simulink model "simQuadrotor"  (R2014b)
settings: Solver=ode45  StartTime=0.0  StopTime=tof  FixedStep=dt  MaxStep=dtmax  RelTol=1e-3
values from neighbouring files (symbols this model uses):
  a = (IzzT - IxxT)./ IxxT    [quadrotor.m]
  alpha = 1    [quadrotor.m]
  Aq = -20    [quadrotor.m]
  Ar = -10*eye(2)    [quadrotor.m]
  Arm = [-20 0 ; 0 -5]    [quadrotor.m]
  As = -50*eye(3)    [quadrotor.m]
  attitudeControlFlag = 4    [quadrotor.m]
  Bq = 1    [quadrotor.m]
  Br = [1 0]    [quadrotor.m]
  Dhat0 = zeros(3,1)    [quadrotor.m]
  Dlimit = 2.5    [quadrotor.m]
  DSecondLimit = 2    [quadrotor.m]
  dtFc = 10e-3    (= 0.01)    [quadrotor.m]
  epsilon = 0.1    [quadrotor.m]
  epsilontheta = 0.1    [quadrotor.m]
  euler0 = [0 0 0]'*pi/180    [quadrotor.m]
  Eulerc_ftc = [0 0 0]'    [quadrotor.m]
  faultyPropellerVec = double(not(faultyPropellerVec))    [quadrotor.m]
  FDstart = 3    [quadrotor.m]
  flims = [0.2*0 3.8*2.5]    [quadrotor.m]
  ftc_f2 = 0.1*2    (= 0.2)    [quadrotor.m]
  g = 9.81    [quadrotor.m]
  GammaW = 10000    [quadrotor.m]
  IxxB = IxxT - 4*IxxP    (= 0.0027)    [quadrotor.m]
  IxxT = 2.7e-3    (= 0.0027)    [quadrotor.m]
  IyyB = IyyT - 4*IyyP    (= 0.0027)    [quadrotor.m]
  IyyT = IxxT    (= 0.0027)    [quadrotor.m]
  IzzB = IzzT - 4*IzzP    (= 0.00514)    [quadrotor.m]
  IzzP = 1.5e-5    (= 1.5e-05)    [quadrotor.m]
  IzzT = 5.2e-3    (= 0.0052)    [quadrotor.m]
  Kdxx = 0.7e-4/10    (= 7e-06)    [quadrotor.m]
  Kdzz = 1.4e-4    (= 0.00014)    [quadrotor.m]
  Kf = 6.41e-6    (= 6.41e-06)    [quadrotor.m]
  Kp = 2*0.75*diag([1 1 1])    [quadrotor.m]
  Kp4 = 0.05    [quadrotor.m]
  Ktau = 1.72e-2    (= 0.0172)    [quadrotor.m]
  Kv = 0*0.005*diag([1 1 1])    [quadrotor.m]
  Kv4 = 0.02    [quadrotor.m]
  l = 0.17    [quadrotor.m]
  m = 0.5    [quadrotor.m]
  nc_ftc = 1    [quadrotor.m]
  nCheby = 3    [quadrotor.m]
  pqr0 = [0 0 0]'*pi/180    [quadrotor.m]
  Ps = lyap(As',Q)    [quadrotor.m]
  q0 = [euler0 ; pqr0]    [quadrotor.m]
  qp0 = 0    [quadrotor.m]
  sigmaMot = 0.015    [quadrotor.m]
  tfault = 5    [quadrotor.m]
  Vb0 = [0 0 0]'    [quadrotor.m]
  W0 = 0    [quadrotor.m]
  Wbnd = 10    [quadrotor.m]
  Xe0 = [0 0 0]'    [quadrotor.m]
  xhat0 = [pqr0]    [quadrotor.m]
undefined symbols (not defined in the file or in its folder): Intmax, Intmin, magnitude, rmax, rmin
libraries: aerolibutil x38, simulink x11, vrlib x3, dspbuff3 x1
(part 3 of 3)

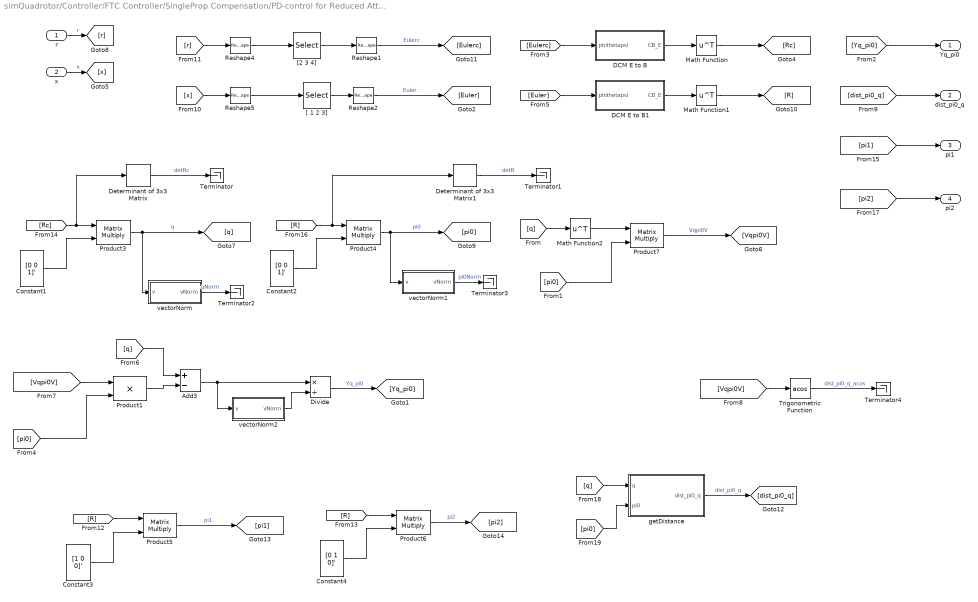
== system simQuadrotor/Controller/FTC Controller/SingleProp Compensation/PD-control for Reduced Attitude-Bullo/getRedAttRelatedPars ==
  r : Inport
  x : Inport  Port=2
  Add3 : Sum  Inputs=+-
  Constant1 : Constant  Value=[0 0 1]'  VectorParams1D=off
  Constant2 : Constant  Value=[0 0 1]'  VectorParams1D=off
  Constant3 : Constant  Value=[1 0 0]'  VectorParams1D=off
  Constant4 : Constant  Value=[0 1 0]'  VectorParams1D=off
  DCM E to B : Subsystem
  DCM E to B1 : Subsystem
  Determinant of 3x3 Matrix : aerolibutil/Determinant of 3x3 Matrix
  Determinant of 3x3 Matrix1 : aerolibutil/Determinant of 3x3 Matrix
  Divide : Product  Inputs=*/
  Math Function : Math  Operator=transpose  SaturateOnIntegerOverflow=on
  Math Function1 : Math  Operator=transpose  SaturateOnIntegerOverflow=on
  Math Function2 : Math  Operator=transpose  SaturateOnIntegerOverflow=on
  Product1 : Product  RndMeth=Zero
  Product{3..7} (5 alike) : Product  Multiplication=Matrix(*)  RndMeth=Zero
  Reshape{1..2,4..5} (4 alike) : Reshape  OutputDimensionality=Column vector (2-D)
  Terminator{,1..4} (5 alike) : Terminator
  Trigonometric Function : Trigonometry  Operator=acos
  "[ 1 2 3]" : Selector  NumberOfDimensions=2  InputPortWidth=3  IndexOptions=Index vector (dialog),Index vector (dialog)  Indices=[1 2 3],1  OutputSizes=1,1
  "[2 3 4]" : Selector  NumberOfDimensions=2  InputPortWidth=3  IndexOptions=Index vector (dialog),Index vector (dialog)  Indices=[2 3 4],1  OutputSizes=1,1
  getDistance : Subsystem
  vectorNorm : Subsystem
  vectorNorm1 : Subsystem
  vectorNorm2 : Subsystem
  Yq_pi0 : Outport
  dist_pi0_q : Outport  Port=2
  pi1 : Outport  Port=3
  pi2 : Outport  Port=4
  wires:
  [pi0] -> getDistance/2(pi0)
  [q] -> getDistance/1(q)
  getDistance/1(dist_pi0_q) -> [dist_pi0_q]  "dist_pi0_q"
  vectorNorm1/1(vNorm) -> Terminator3/1  "pi0Norm"
  vectorNorm/1(vNorm) -> Terminator2/1  "qNorm"
  Determinant of 3x3 Matrix1/1 -> Terminator1/1  "detR"
  Determinant of 3x3 Matrix/1 -> Terminator/1  "detRc"
  [pi2] -> pi2/1
  [pi1] -> pi1/1
  [R] -> Product6/1
  Constant4/1 -> Product6/2
  Product6/1 -> [pi2]  "pi2"
  [R] -> Product5/1
  Constant3/1 -> Product5/2
  Product5/1 -> [pi1]  "pi1"
  [Yq_pi0] -> Yq_pi0/1
  Trigonometric Function/1 -> Terminator4/1  "dist_pi0_q_acos"
  [Vqpi0V] -> Trigonometric Function/1
  [Vqpi0V] -> Product1/1
  Product7/1 -> [Vqpi0V]  "Vqpi0V"
  Divide/1 -> [Yq_pi0]  "Yq_pi0"
  vectorNorm2/1(vNorm) -> Divide/2
  Add3/1 -> Divide/1, vectorNorm2/1(v)
  Product1/1 -> Add3/2
  [q] -> Add3/1
  [pi0] -> Product1/2
  [pi0] -> Product7/2
  Math Function2/1 -> Product7/1
  [q] -> Math Function2/1
  [dist_pi0_q] -> dist_pi0_q/1
  [Rc] -> Product3/1, Determinant of 3x3 Matrix/1
  Constant1/1 -> Product3/2
  Product3/1 -> [q], vectorNorm/1(v)  "q"
  [R] -> Product4/1, Determinant of 3x3 Matrix1/1
  Constant2/1 -> Product4/2
  Product4/1 -> [pi0], vectorNorm1/1(v)  "pi0"
  r/1 -> [r]  "r"
  x/1 -> [x]  "x"
  Math Function1/1 -> [R]
  [x] -> Reshape5/1
  Math Function/1 -> [Rc]
  "[ 1 2 3]"/1 -> Reshape2/1
  Reshape5/1 -> "[ 1 2 3]"/1
  Reshape2/1 -> [Euler]  "Euler"
  Reshape1/1 -> [Eulerc]  "Eulerc"
  "[2 3 4]"/1 -> Reshape1/1
  [r] -> Reshape4/1
  [Eulerc] -> DCM E to B/1(phithetapsi)
  DCM E to B/1(CB_E) -> Math Function/1
  Reshape4/1 -> "[2 3 4]"/1
  [Euler] -> DCM E to B1/1(phithetapsi)
  DCM E to B1/1(CB_E) -> Math Function1/1

== system simQuadrotor/Controller/FTC Controller/SingleProp Compensation/Perturbation Calculation/Reference model ==
  x1 : Inport
  Gain : Gain  Gain=Arm  Multiplication=Matrix(K*u)
  f1r : Outport
  wires:
  Gain/1 -> [f1r]
  x1/1 -> [x1]
  [x1] -> Gain/1
  [f1r] -> f1r/1

== system simQuadrotor/Controller/FTC Controller/SingleProp Compensation/Perturbation Calculation/System model ==
  x1 : Inport
  w3 : Inport  Port=2
  r : Inport  Port=3
  p1p : Inport  Port=4
  p2p : Inport  Port=5
  Add2 : Sum  Inputs=+++
  Constant : Constant  Value=a  VectorParams1D=off
  Constant1 : Constant  Value=Br  VectorParams1D=off
  Constant2 : Constant  Value=ftc_f2  VectorParams1D=off
  Constant3 : Constant  Value=[0 0]'  VectorParams1D=off
  Constant5 : Constant  Value=0  VectorParams1D=off
  Gain : Gain  Gain=-1
  Gain1 : Gain
  Gain2 : Gain  Gain=l/IxxT
  Gain3 : Gain  Gain=[0 ; 1]  Multiplication=Matrix(K*u)
  Gain4 : Gain  Gain=-1
  Mux : Mux  Inputs=2
  Product1 : Product  Multiplication=Matrix(*)
  Product2 : Product
  Product3 : Product  Multiplication=Matrix(*)
  Product4 : Product  Multiplication=Matrix(*)
  Reshape : Reshape  OutputDimensionality=Customize  OutputDimensions=[2,2]
  Reshape3 : Reshape  OutputDimensionality=Column vector (2-D)
  Vector Concatenate : Concatenate  NumInputs=3
  f1 : Outport
  wires:
  Constant5/1 -> Vector Concatenate/3
  Gain1/1 -> Vector Concatenate/2
  Vector Concatenate/1 -> Reshape/1
  [p2p] -> Gain1/1
  Constant3/1 -> Vector Concatenate/1
  p2p/1 -> [p2p]
  p1p/1 -> [p1p]
  Product4/1 -> Add2/2
  Product3/1 -> Add2/1
  [r] -> Product4/2
  Product1/1 -> Product4/1
  [Br] -> Product1/2
  Reshape3/1 -> Product1/1
  [x1] -> Product3/2
  Reshape/1 -> Product3/1
  [p1p] -> Gain4/1
  Mux/1 -> Reshape3/1
  Constant1/1 -> [Br]
  w3/1 -> [w3]
  r/1 -> [r]
  [a] -> Product2/1  "a"
  [w3] -> Product2/2
  Add2/1 -> [f1]
  Product2/1 -> Gain/1  "aw3"
  Constant/1 -> [a]
  x1/1 -> [x1]
  [f1] -> f1/1
  Gain/1 -> Mux/2
  Constant2/1 -> Gain2/1
  Gain2/1 -> Gain3/1
  Gain3/1 -> Add2/3  "d"
  Gain4/1 -> Mux/1

== system simQuadrotor/Controller/FTC Controller/SingleProp Compensation/Perturbation Calculation/getStates ==
  x : Inport
  Constant : Constant  Value=[0 0 1]'  VectorParams1D=off
  Mux : Mux  Inputs=2
  Reshape{1,3..4,6..7} (5 alike) : Reshape  OutputDimensionality=Column vector (2-D)
  "[2 3 4]1" : Selector  InputPortWidth=3
  "[2 3 4]2" : Selector  InputPortWidth=3  Indices=2
  "[2 3 4]3" : Selector  InputPortWidth=3  Indices=3
  "[4 5 6]" : Selector  NumberOfDimensions=2  InputPortWidth=3  IndexOptions=Index vector (dialog),Index vector (dialog)  Indices=[4 5 6],1  OutputSizes=1,1
  calcParameters : Subsystem  TreatAsAtomicUnit=on
  getDistance : Subsystem
  x1 : Outport
  x2 : Outport  Port=2
  w3 : Outport  Port=3
  p1p : Outport  Port=4
  p2p : Outport  Port=5
  wires:
  [p2p] -> p2p/1
  [p1p] -> p1p/1
  "[2 3 4]1"/1 -> Mux/2
  calcParameters/3(p) -> [p]  "p"
  [p] -> getDistance/2(p)
  Constant/1 -> getDistance/1(q)
  getDistance/1(dist) -> [dist]  "dist"
  calcParameters/2(p2p) -> [p2p]  "p2p"
  calcParameters/1(p1p) -> [p1p]  "p1p"
  [x] -> calcParameters/1(x)
  Reshape7/1 -> [w3]
  Reshape6/1 -> [x2]
  Reshape3/1 -> [x1]
  "[2 3 4]3"/1 -> Reshape7/1
  [w] -> "[2 3 4]3"/1
  "[2 3 4]2"/1 -> Reshape6/1
  [w3] -> w3/1
  [w] -> "[2 3 4]2"/1
  Mux/1 -> Reshape3/1
  [dist] -> Mux/1
  [w] -> "[2 3 4]1"/1
  [x2] -> x2/1  "x2"
  [x1] -> x1/1  "x1"
  x/1 -> [x]  "x"
  Reshape1/1 -> [w]  "w"
  "[4 5 6]"/1 -> Reshape1/1
  [x] -> Reshape4/1
  Reshape4/1 -> "[4 5 6]"/1

== system simQuadrotor/Controller/Nominal Controller/PD-Attitude Control with wB_IB/get eR/DCM E to B ==
  phithetapsi : Inport
  Create 3x3 Matrix : aerolibutil/Create 3x3 Matrix
  Fcn11 : Fcn  Expr=u(5)*u(6)
  Fcn12 : Fcn  Expr=u(3)*u(5)
  Fcn13 : Fcn  Expr=-u(2)
  Fcn21 : Fcn  Expr=u(1)*u(2)*u(6)-u(4)*u(3)
  Fcn22 : Fcn  Expr=u(1)*u(2)*u(3)+u(4)*u(6)
  Fcn23 : Fcn  Expr=u(1)*u(5)
  Fcn31 : Fcn  Expr=u(4)*u(2)*u(6)+u(1)*u(3)
  Fcn32 : Fcn  Expr=u(4)*u(2)*u(3)-u(1)*u(6)
  Fcn33 : Fcn  Expr=u(4)*u(5)
  Mux : Mux  Inputs=2
  sincos : Trigonometry  Operator=sincos
  CB_E : Outport
  wires:
  Create 3x3 Matrix/1 -> CB_E/1  "CB_E"
  phithetapsi/1 -> sincos/1  "phithetapsi"
  Fcn33/1 -> Create 3x3 Matrix/9
  Fcn32/1 -> Create 3x3 Matrix/8
  Fcn23/1 -> Create 3x3 Matrix/6
  Fcn22/1 -> Create 3x3 Matrix/5
  Fcn31/1 -> Create 3x3 Matrix/7
  Fcn21/1 -> Create 3x3 Matrix/4
  Fcn13/1 -> Create 3x3 Matrix/3
  Fcn12/1 -> Create 3x3 Matrix/2
  Fcn11/1 -> Create 3x3 Matrix/1
  Mux/1 -> Fcn21/1, Fcn13/1, Fcn12/1, Fcn11/1, Fcn22/1, Fcn23/1, Fcn31/1, Fcn33/1, Fcn32/1
  sincos/2 -> Mux/2
  sincos/1 -> Mux/1

== system simQuadrotor/Controller/Nominal Controller/PD-Attitude Control with wB_IB/get eR/DCM E to B1 ==
  phithetapsi : Inport
  Create 3x3 Matrix : aerolibutil/Create 3x3 Matrix
  Fcn11 : Fcn  Expr=u(5)*u(6)
  Fcn12 : Fcn  Expr=u(3)*u(5)
  Fcn13 : Fcn  Expr=-u(2)
  Fcn21 : Fcn  Expr=u(1)*u(2)*u(6)-u(4)*u(3)
  Fcn22 : Fcn  Expr=u(1)*u(2)*u(3)+u(4)*u(6)
  Fcn23 : Fcn  Expr=u(1)*u(5)
  Fcn31 : Fcn  Expr=u(4)*u(2)*u(6)+u(1)*u(3)
  Fcn32 : Fcn  Expr=u(4)*u(2)*u(3)-u(1)*u(6)
  Fcn33 : Fcn  Expr=u(4)*u(5)
  Mux : Mux  Inputs=2
  sincos : Trigonometry  Operator=sincos
  CB_E : Outport
  wires:
  Create 3x3 Matrix/1 -> CB_E/1  "CB_E"
  phithetapsi/1 -> sincos/1  "phithetapsi"
  Fcn33/1 -> Create 3x3 Matrix/9
  Fcn32/1 -> Create 3x3 Matrix/8
  Fcn23/1 -> Create 3x3 Matrix/6
  Fcn22/1 -> Create 3x3 Matrix/5
  Fcn31/1 -> Create 3x3 Matrix/7
  Fcn21/1 -> Create 3x3 Matrix/4
  Fcn13/1 -> Create 3x3 Matrix/3
  Fcn12/1 -> Create 3x3 Matrix/2
  Fcn11/1 -> Create 3x3 Matrix/1
  Mux/1 -> Fcn21/1, Fcn13/1, Fcn12/1, Fcn11/1, Fcn22/1, Fcn23/1, Fcn31/1, Fcn33/1, Fcn32/1
  sincos/2 -> Mux/2
  sincos/1 -> Mux/1

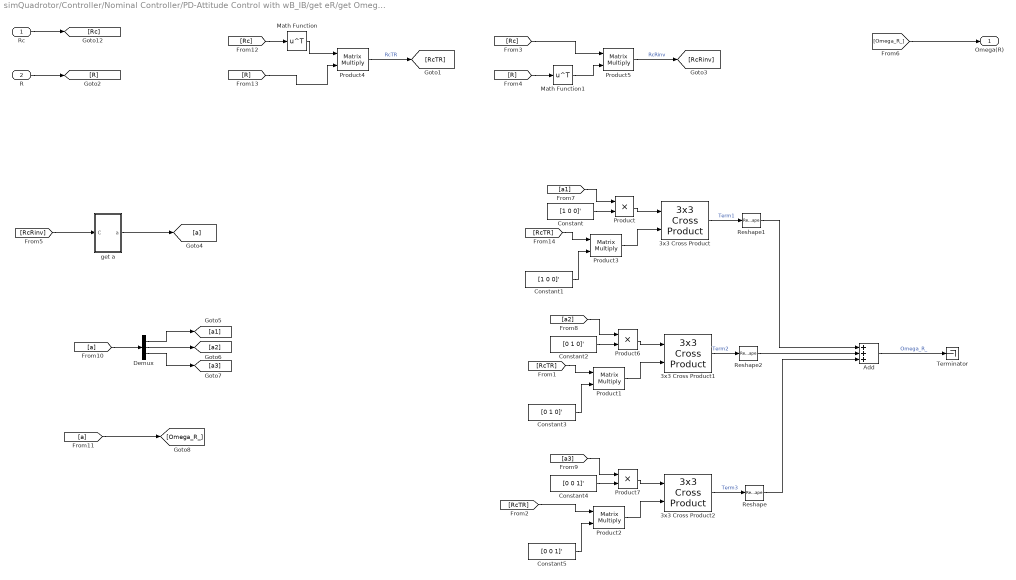
== system simQuadrotor/Controller/Nominal Controller/PD-Attitude Control with wB_IB/get eR/get Omega(R) RBAC ==
  Rc : Inport
  R : Inport  Port=2
  3x3 Cross Product : aerolibutil/3x3 Cross Product
  3x3 Cross Product1 : aerolibutil/3x3 Cross Product
  3x3 Cross Product2 : aerolibutil/3x3 Cross Product
  Add : Sum  Inputs=+++
  Constant : Constant  Value=[1 0 0]'  VectorParams1D=off
  Constant1 : Constant  Value=[1 0 0]'  VectorParams1D=off
  Constant2 : Constant  Value=[0 1 0]'  VectorParams1D=off
  Constant3 : Constant  Value=[0 1 0]'  VectorParams1D=off
  Constant4 : Constant  Value=[0 0 1]'  VectorParams1D=off
  Constant5 : Constant  Value=[0 0 1]'  VectorParams1D=off
  Demux : Demux  Outputs=3
  Math Function : Math  Operator=transpose  SaturateOnIntegerOverflow=on
  Math Function1 : Math  Operator=transpose  SaturateOnIntegerOverflow=on
  Product : Product  RndMeth=Zero
  Product{1..5} (5 alike) : Product  Multiplication=Matrix(*)  RndMeth=Zero
  Product6 : Product  RndMeth=Zero
  Product7 : Product  RndMeth=Zero
  Reshape : Reshape  OutputDimensionality=Column vector (2-D)
  Reshape1 : Reshape  OutputDimensionality=Column vector (2-D)
  Reshape2 : Reshape  OutputDimensionality=Column vector (2-D)
  Terminator : Terminator
  get a : Subsystem
  Omega(R) : Outport
  wires:
  [a] -> [Omega_R_]
  Reshape/1 -> Add/3
  Reshape2/1 -> Add/2
  Reshape1/1 -> Add/1
  Demux/3 -> [a3]
  Demux/2 -> [a2]
  Demux/1 -> [a1]
  [a] -> Demux/1
  [a3] -> Product7/1
  [a2] -> Product6/1
  [a1] -> Product/1
  get a/1(a) -> [a]
  [RcRinv] -> get a/1(C)
  Math Function1/1 -> Product5/2
  Product5/1 -> [RcRinv]  "RcRinv"
  [R] -> Math Function1/1
  [Rc] -> Product5/1
  R/1 -> [R]
  Rc/1 -> [Rc]
  Math Function/1 -> Product4/1
  Product4/1 -> [RcTR]  "RcTR"
  [R] -> Product4/2
  [Rc] -> Math Function/1
  [Omega_R_] -> Omega(R)/1
  Add/1 -> Terminator/1  "Omega_R_"
  3x3 Cross Product2/1 -> Reshape/1  "Term3"
  3x3 Cross Product1/1 -> Reshape2/1  "Term2"
  3x3 Cross Product/1 -> Reshape1/1  "Term1"
  Product7/1 -> 3x3 Cross Product2/1
  Product2/1 -> 3x3 Cross Product2/2
  Constant5/1 -> Product2/2
  [RcTR] -> Product2/1
  Constant4/1 -> Product7/2
  Product6/1 -> 3x3 Cross Product1/1
  Product/1 -> 3x3 Cross Product/1
  Product1/1 -> 3x3 Cross Product1/2
  Constant3/1 -> Product1/2
  [RcTR] -> Product1/1
  Constant2/1 -> Product6/2
  Product3/1 -> 3x3 Cross Product/2
  Constant1/1 -> Product3/2
  [RcTR] -> Product3/1
  Constant/1 -> Product/2

== system simQuadrotor/Controller/Nominal Controller/PD-Attitude Control with wB_IB/get eR/get eR ==
  note: Vee map
  Rc : Inport
  R : Inport  Port=2
  13 : Selector  NumberOfDimensions=2  InputPortWidth=3  IndexOptions=Index vector (dialog),Index vector (dialog)  Indices=1,3  OutputSizes=1,1
  21 : Selector  NumberOfDimensions=2  InputPortWidth=3  IndexOptions=Index vector (dialog),Index vector (dialog)  Indices=2,1  OutputSizes=1,1
  32 : Selector  NumberOfDimensions=2  InputPortWidth=3  IndexOptions=Index vector (dialog),Index vector (dialog)  Indices=3,2  OutputSizes=1,1
  Add : Sum  Inputs=+-
  Gain4 : Gain  Gain=1/2
  Math Function1 : Math  Operator=transpose  SaturateOnIntegerOverflow=on
  Math Function2 : Math  Operator=transpose  SaturateOnIntegerOverflow=on
  Math Function3 : Math  Operator=transpose  SaturateOnIntegerOverflow=on
  Mux : Mux  Inputs=3
  Product : Product  RndMeth=Zero
  Product1 : Product  Multiplication=Matrix(*)  RndMeth=Zero
  Product2 : Product  Multiplication=Matrix(*)  RndMeth=Zero
  Product5 : Product  Multiplication=Matrix(*)  RndMeth=Zero
  Reshape6 : Reshape  OutputDimensionality=Column vector (2-D)
  get alpha : Subsystem
  eR : Outport
  wires:
  Product/1 -> [eR]
  [alpha] -> Product/2
  Reshape6/1 -> Product/1  "eR_non"
  [Rc] -> Math Function2/1
  Math Function2/1 -> Product1/1
  [R] -> Product1/2
  [R] -> Math Function3/1
  Math Function3/1 -> Product2/1
  [Rc] -> Product2/2
  Product1/1 -> Add/1  "RcTR"
  Product2/1 -> Add/2  "RTRc"
  Add/1 -> Gain4/1
  Gain4/1 -> 32/1, 21/1, 13/1
  32/1 -> Mux/1
  13/1 -> Mux/2
  21/1 -> Mux/3
  Mux/1 -> Reshape6/1
  [RcRinv] -> get alpha/1(C)
  get alpha/1(alpha) -> [alpha]  "alpha"
  [eR] -> eR/1
  Rc/1 -> [Rc]
  R/1 -> [R]
  [Rc] -> Product5/1
  [R] -> Math Function1/1
  Product5/1 -> [RcRinv]  "RcRinv"
  Math Function1/1 -> Product5/2

== system simQuadrotor/Controller/Nominal Controller/PD-control for Attitude/get Omega(R) RBAC/get a ==
  C : Inport
  11 : Selector  NumberOfDimensions=2  InputPortWidth=3  IndexOptions=Index vector (dialog),Index vector (dialog)  Indices=1,1  OutputSizes=1,1
  12 : Selector  NumberOfDimensions=2  InputPortWidth=3  IndexOptions=Index vector (dialog),Index vector (dialog)  Indices=1,2  OutputSizes=1,1
  13 : Selector  NumberOfDimensions=2  InputPortWidth=3  IndexOptions=Index vector (dialog),Index vector (dialog)  Indices=1,3  OutputSizes=1,1
  21 : Selector  NumberOfDimensions=2  InputPortWidth=3  IndexOptions=Index vector (dialog),Index vector (dialog)  Indices=2,1  OutputSizes=1,1
  22 : Selector  NumberOfDimensions=2  InputPortWidth=3  IndexOptions=Index vector (dialog),Index vector (dialog)  Indices=2,2  OutputSizes=1,1
  23 : Selector  NumberOfDimensions=2  InputPortWidth=3  IndexOptions=Index vector (dialog),Index vector (dialog)  Indices=2,3  OutputSizes=1,1
  31 : Selector  NumberOfDimensions=2  InputPortWidth=3  IndexOptions=Index vector (dialog),Index vector (dialog)  Indices=3,1  OutputSizes=1,1
  32 : Selector  NumberOfDimensions=2  InputPortWidth=3  IndexOptions=Index vector (dialog),Index vector (dialog)  Indices=3,2  OutputSizes=1,1
  33 : Selector  NumberOfDimensions=2  InputPortWidth=3  IndexOptions=Index vector (dialog),Index vector (dialog)  Indices=3,3  OutputSizes=1,1
  Add : Sum  Inputs=+++-
  Add1 : Sum  Inputs=+-
  Add2 : Sum  Inputs=+-
  Add3 : Sum  Inputs=+-
  Constant5 : Constant
  Divide : Product  Inputs=*/
  Gain1 : Gain  Gain=0.5
  Gain2 : Gain  Gain=2
  Gain3 : Gain
  Mux : Mux  Inputs=3
  Product : Product  RndMeth=Zero
  Trigonometric Function : Trigonometry  Operator=acos
  Trigonometric Function1 : Trigonometry
  a : Outport
  wires:
  [alpha] -> Product/2
  Product/1 -> Gain3/1
  Divide/1 -> Product/1
  Gain3/1 -> [a]  "a"
  [a] -> a/1
  Gain2/1 -> Divide/2
  Mux/1 -> Divide/1
  [sinAlpha] -> Gain2/1
  Add3/1 -> Mux/3
  Add2/1 -> Mux/2
  Add1/1 -> Mux/1
  [C21] -> Add3/2
  [C12] -> Add3/1
  [C13] -> Add2/2
  [C31] -> Add2/1
  [C32] -> Add1/2
  [C23] -> Add1/1
  Trigonometric Function1/1 -> [sinAlpha]
  [alpha] -> Trigonometric Function1/1
  Trigonometric Function/1 -> [alpha]  "alpha"
  Gain1/1 -> Trigonometric Function/1
  Add/1 -> Gain1/1
  Constant5/1 -> Add/4
  [C33] -> Add/3
  [C22] -> Add/2
  [C11] -> Add/1
  33/1 -> [C33]
  32/1 -> [C32]
  31/1 -> [C31]
  23/1 -> [C23]
  22/1 -> [C22]
  21/1 -> [C21]
  13/1 -> [C13]
  12/1 -> [C12]
  11/1 -> [C11]
  C/1 -> 11/1, 12/1, 13/1, 21/1, 22/1, 23/1, 31/1, 32/1, 33/1

== system simQuadrotor/Controller/Nominal Controller/PD-control for Attitude/get eR/get alpha ==
  C : Inport
  11 : Selector  NumberOfDimensions=2  InputPortWidth=3  IndexOptions=Index vector (dialog),Index vector (dialog)  Indices=1,1  OutputSizes=1,1
  22 : Selector  NumberOfDimensions=2  InputPortWidth=3  IndexOptions=Index vector (dialog),Index vector (dialog)  Indices=2,2  OutputSizes=1,1
  33 : Selector  NumberOfDimensions=2  InputPortWidth=3  IndexOptions=Index vector (dialog),Index vector (dialog)  Indices=3,3  OutputSizes=1,1
  Add : Sum  Inputs=+++-
  Constant5 : Constant
  Gain1 : Gain  Gain=0.5
  Trigonometric Function : Trigonometry  Operator=acos
  alpha : Outport
  wires:
  C/1 -> 33/1, 11/1, 22/1
  11/1 -> [C11]
  22/1 -> [C22]
  33/1 -> [C33]
  [C11] -> Add/1
  [C22] -> Add/2
  [C33] -> Add/3
  Constant5/1 -> Add/4
  Add/1 -> Gain1/1
  Gain1/1 -> Trigonometric Function/1
  Trigonometric Function/1 -> [alpha]  "alpha"
  [alpha] -> alpha/1

== system simQuadrotor/Controller/Nominal Controller/PD-control for AttitudeAlt/get Omega(R) RBAC/get a ==
  R : Inport
  Rc : Inport  Port=2
  3x3 Cross Product1 : aerolibutil/3x3 Cross Product
  Constant : Constant  Value=[0 0 1]'  VectorParams1D=off
  Constant1 : Constant  Value=[0 0 1]'  VectorParams1D=off
  Divide1 : Product  Inputs=*/
  Divide2 : Product  Multiplication=Matrix(*)
  Math Function : Math  Operator=transpose  SaturateOnIntegerOverflow=on
  Product1 : Product  Multiplication=Matrix(*)  RndMeth=Zero
  Product2 : Product  Multiplication=Matrix(*)  RndMeth=Zero
  Reshape : Reshape  OutputDimensionality=Column vector (2-D)
  Sqrt : Sqrt  SaturateOnIntegerOverflow=on
  a : Outport
  wires:
  [a] -> a/1
  Rc/1 -> [Rc]
  R/1 -> [R]
  [R] -> Product1/1
  Constant/1 -> Product1/2
  Product1/1 -> [G]
  [Rc] -> Product2/1
  Constant1/1 -> Product2/2
  Product2/1 -> [Gc]
  [G] -> 3x3 Cross Product1/1
  [Gc] -> 3x3 Cross Product1/2
  3x3 Cross Product1/1 -> [A1]
  [A1] -> Reshape/1, Math Function/1, Divide1/1
  Math Function/1 -> Divide2/1
  Divide2/1 -> Sqrt/1
  Sqrt/1 -> Divide1/2
  Divide1/1 -> [a]
  Reshape/1 -> Divide2/2

== system simQuadrotor/Controller/Nominal Controller/PD-control for AttitudeAlt/get Omega(R) RBAC/get a1_old ==
  C : Inport
  11 : Selector  NumberOfDimensions=2  InputPortWidth=3  IndexOptions=Index vector (dialog),Index vector (dialog)  Indices=1,1  OutputSizes=1,1
  12 : Selector  NumberOfDimensions=2  InputPortWidth=3  IndexOptions=Index vector (dialog),Index vector (dialog)  Indices=1,2  OutputSizes=1,1
  13 : Selector  NumberOfDimensions=2  InputPortWidth=3  IndexOptions=Index vector (dialog),Index vector (dialog)  Indices=1,3  OutputSizes=1,1
  21 : Selector  NumberOfDimensions=2  InputPortWidth=3  IndexOptions=Index vector (dialog),Index vector (dialog)  Indices=2,1  OutputSizes=1,1
  22 : Selector  NumberOfDimensions=2  InputPortWidth=3  IndexOptions=Index vector (dialog),Index vector (dialog)  Indices=2,2  OutputSizes=1,1
  23 : Selector  NumberOfDimensions=2  InputPortWidth=3  IndexOptions=Index vector (dialog),Index vector (dialog)  Indices=2,3  OutputSizes=1,1
  31 : Selector  NumberOfDimensions=2  InputPortWidth=3  IndexOptions=Index vector (dialog),Index vector (dialog)  Indices=3,1  OutputSizes=1,1
  32 : Selector  NumberOfDimensions=2  InputPortWidth=3  IndexOptions=Index vector (dialog),Index vector (dialog)  Indices=3,2  OutputSizes=1,1
  33 : Selector  NumberOfDimensions=2  InputPortWidth=3  IndexOptions=Index vector (dialog),Index vector (dialog)  Indices=3,3  OutputSizes=1,1
  Add : Sum  Inputs=+++-
  Add1 : Sum  Inputs=+-
  Add2 : Sum  Inputs=+-
  Add3 : Sum  Inputs=+-
  Constant5 : Constant
  Divide : Product  Inputs=*/
  Gain1 : Gain  Gain=0.5
  Gain2 : Gain  Gain=2
  Gain3 : Gain
  Mux : Mux  Inputs=3
  Product : Product  RndMeth=Zero
  Trigonometric Function : Trigonometry  Operator=acos
  Trigonometric Function1 : Trigonometry
  a : Outport
  wires:
  [alpha] -> Product/2
  Product/1 -> Gain3/1
  Divide/1 -> Product/1
  Gain3/1 -> [a]  "a"
  [a] -> a/1
  Gain2/1 -> Divide/2
  Mux/1 -> Divide/1
  [sinAlpha] -> Gain2/1
  Add3/1 -> Mux/3
  Add2/1 -> Mux/2
  Add1/1 -> Mux/1
  [C21] -> Add3/2
  [C12] -> Add3/1
  [C13] -> Add2/2
  [C31] -> Add2/1
  [C32] -> Add1/2
  [C23] -> Add1/1
  Trigonometric Function1/1 -> [sinAlpha]
  [alpha] -> Trigonometric Function1/1
  Trigonometric Function/1 -> [alpha]  "alpha"
  Gain1/1 -> Trigonometric Function/1
  Add/1 -> Gain1/1
  Constant5/1 -> Add/4
  [C33] -> Add/3
  [C22] -> Add/2
  [C11] -> Add/1
  33/1 -> [C33]
  32/1 -> [C32]
  31/1 -> [C31]
  23/1 -> [C23]
  22/1 -> [C22]
  21/1 -> [C21]
  13/1 -> [C13]
  12/1 -> [C12]
  11/1 -> [C11]
  C/1 -> 11/1, 12/1, 13/1, 21/1, 22/1, 23/1, 31/1, 32/1, 33/1

== system simQuadrotor/Controller/Nominal Controller/PD-control for AttitudeAlt/get eR/get alpha ==
  C : Inport
  11 : Selector  NumberOfDimensions=2  InputPortWidth=3  IndexOptions=Index vector (dialog),Index vector (dialog)  Indices=1,1  OutputSizes=1,1
  22 : Selector  NumberOfDimensions=2  InputPortWidth=3  IndexOptions=Index vector (dialog),Index vector (dialog)  Indices=2,2  OutputSizes=1,1
  33 : Selector  NumberOfDimensions=2  InputPortWidth=3  IndexOptions=Index vector (dialog),Index vector (dialog)  Indices=3,3  OutputSizes=1,1
  Add : Sum  Inputs=+++-
  Constant5 : Constant
  Gain1 : Gain  Gain=0.5
  Trigonometric Function : Trigonometry  Operator=acos
  alpha : Outport
  wires:
  [alpha] -> alpha/1
  Trigonometric Function/1 -> [alpha]  "alpha"
  Gain1/1 -> Trigonometric Function/1
  Add/1 -> Gain1/1
  Constant5/1 -> Add/4
  [C33] -> Add/3
  [C22] -> Add/2
  [C11] -> Add/1
  33/1 -> [C33]
  22/1 -> [C22]
  11/1 -> [C11]
  C/1 -> 22/1, 11/1, 33/1

== system simQuadrotor/Controller/Nominal Controller/PD-control for Reduced Attitude-Bullo/getRedAttRelatedPars/DCM E to B ==
  phithetapsi : Inport
  Create 3x3 Matrix : aerolibutil/Create 3x3 Matrix
  Fcn11 : Fcn  Expr=u(5)*u(6)
  Fcn12 : Fcn  Expr=u(3)*u(5)
  Fcn13 : Fcn  Expr=-u(2)
  Fcn21 : Fcn  Expr=u(1)*u(2)*u(6)-u(4)*u(3)
  Fcn22 : Fcn  Expr=u(1)*u(2)*u(3)+u(4)*u(6)
  Fcn23 : Fcn  Expr=u(1)*u(5)
  Fcn31 : Fcn  Expr=u(4)*u(2)*u(6)+u(1)*u(3)
  Fcn32 : Fcn  Expr=u(4)*u(2)*u(3)-u(1)*u(6)
  Fcn33 : Fcn  Expr=u(4)*u(5)
  Mux : Mux  Inputs=2
  sincos : Trigonometry  Operator=sincos
  CB_E : Outport
  wires:
  sincos/1 -> Mux/1
  sincos/2 -> Mux/2
  Mux/1 -> Fcn32/1, Fcn33/1, Fcn31/1, Fcn23/1, Fcn22/1, Fcn11/1, Fcn12/1, Fcn13/1, Fcn21/1
  Fcn11/1 -> Create 3x3 Matrix/1
  Fcn12/1 -> Create 3x3 Matrix/2
  Fcn13/1 -> Create 3x3 Matrix/3
  Fcn21/1 -> Create 3x3 Matrix/4
  Fcn31/1 -> Create 3x3 Matrix/7
  Fcn22/1 -> Create 3x3 Matrix/5
  Fcn23/1 -> Create 3x3 Matrix/6
  Fcn32/1 -> Create 3x3 Matrix/8
  Fcn33/1 -> Create 3x3 Matrix/9
  phithetapsi/1 -> sincos/1  "phithetapsi"
  Create 3x3 Matrix/1 -> CB_E/1  "CB_E"

== system simQuadrotor/Controller/Nominal Controller/PD-control for Reduced Attitude-Bullo/getRedAttRelatedPars/DCM E to B1 ==
  phithetapsi : Inport
  Create 3x3 Matrix : aerolibutil/Create 3x3 Matrix
  Fcn11 : Fcn  Expr=u(5)*u(6)
  Fcn12 : Fcn  Expr=u(3)*u(5)
  Fcn13 : Fcn  Expr=-u(2)
  Fcn21 : Fcn  Expr=u(1)*u(2)*u(6)-u(4)*u(3)
  Fcn22 : Fcn  Expr=u(1)*u(2)*u(3)+u(4)*u(6)
  Fcn23 : Fcn  Expr=u(1)*u(5)
  Fcn31 : Fcn  Expr=u(4)*u(2)*u(6)+u(1)*u(3)
  Fcn32 : Fcn  Expr=u(4)*u(2)*u(3)-u(1)*u(6)
  Fcn33 : Fcn  Expr=u(4)*u(5)
  Mux : Mux  Inputs=2
  sincos : Trigonometry  Operator=sincos
  CB_E : Outport
  wires:
  sincos/1 -> Mux/1
  sincos/2 -> Mux/2
  Mux/1 -> Fcn32/1, Fcn33/1, Fcn31/1, Fcn23/1, Fcn22/1, Fcn11/1, Fcn12/1, Fcn13/1, Fcn21/1
  Fcn11/1 -> Create 3x3 Matrix/1
  Fcn12/1 -> Create 3x3 Matrix/2
  Fcn13/1 -> Create 3x3 Matrix/3
  Fcn21/1 -> Create 3x3 Matrix/4
  Fcn31/1 -> Create 3x3 Matrix/7
  Fcn22/1 -> Create 3x3 Matrix/5
  Fcn23/1 -> Create 3x3 Matrix/6
  Fcn32/1 -> Create 3x3 Matrix/8
  Fcn33/1 -> Create 3x3 Matrix/9
  phithetapsi/1 -> sincos/1  "phithetapsi"
  Create 3x3 Matrix/1 -> CB_E/1  "CB_E"

== system simQuadrotor/Controller/Nominal Controller/PD-control for Reduced Attitude-Bullo/getRedAttRelatedPars/getDistance ==
  q : Inport
  pi0 : Inport  Port=2
  3x3 Cross Product1 : aerolibutil/3x3 Cross Product
  Trigonometric Function : Trigonometry  Operator=asin
  vectorNorm : Subsystem
  dist_pi0_q : Outport
  wires:
  [q] -> 3x3 Cross Product1/2
  [pi0] -> 3x3 Cross Product1/1
  3x3 Cross Product1/1 -> vectorNorm/1(v)
  [dist_pi0_q] -> dist_pi0_q/1
  pi0/1 -> [pi0]
  q/1 -> [q]
  Trigonometric Function/1 -> [dist_pi0_q]
  vectorNorm/1(vNorm) -> Trigonometric Function/1

== system simQuadrotor/Controller/Nominal Controller/PD-control for Reduced Attitude-Bullo/getRedAttRelatedPars/vectorNorm ==
  v : Inport
  Math Function4 : Math  Operator=transpose  SaturateOnIntegerOverflow=on
  Product8 : Product  Multiplication=Matrix(*)  RndMeth=Zero
  Sqrt1 : Sqrt  SaturateOnIntegerOverflow=on
  vNorm : Outport
  wires:
  Sqrt1/1 -> vNorm/1
  v/1 -> Product8/2, Math Function4/1
  Product8/1 -> Sqrt1/1
  Math Function4/1 -> Product8/1

== system simQuadrotor/Controller/Nominal Controller/PD-control for Reduced Attitude-Bullo/getRedAttRelatedPars/vectorNorm1 ==
  v : Inport
  Math Function4 : Math  Operator=transpose  SaturateOnIntegerOverflow=on
  Product8 : Product  Multiplication=Matrix(*)  RndMeth=Zero
  Sqrt1 : Sqrt  SaturateOnIntegerOverflow=on
  vNorm : Outport
  wires:
  Math Function4/1 -> Product8/1
  Product8/1 -> Sqrt1/1
  v/1 -> Math Function4/1, Product8/2
  Sqrt1/1 -> vNorm/1

== system simQuadrotor/Controller/Nominal Controller/PD-control for Reduced Attitude-Bullo/getRedAttRelatedPars/vectorNorm2 ==
  v : Inport
  Math Function4 : Math  Operator=transpose  SaturateOnIntegerOverflow=on
  Product8 : Product  Multiplication=Matrix(*)  RndMeth=Zero
  Sqrt1 : Sqrt  SaturateOnIntegerOverflow=on
  vNorm : Outport
  wires:
  Math Function4/1 -> Product8/1
  Product8/1 -> Sqrt1/1
  v/1 -> Math Function4/1, Product8/2
  Sqrt1/1 -> vNorm/1

== system simQuadrotor/Controller/Disturbance Estimator/getDisturbance/Chebyshev Basis Functions/Chebyshev Polynomail Value Calculation/If Action Subsystem ==
  x : Inport
  polyvals : Inport  Port=2
  Action Port : ActionPort  PropagateVarSize=During execution  ActionType=then
  Add : Sum  Inputs=+-
  Constant : Constant  Value=nCheby
  Constant1 : Constant  Value=nCheby-1
  Gain : Gain  Gain=2
  Product : Product  RndMeth=Zero
  Selector : Selector  IndexOptions=Index vector (port)  Indices=[1 3]
  Selector1 : Selector  IndexOptions=Index vector (port)  Indices=[1 3]
  polyval : Outport
  wires:
  x/1 -> [x]
  polyvals/1 -> [polyvals]  "if.polyvals"
  [polyvals] -> Selector/1
  Constant1/1 -> Selector/2
  Selector/1 -> [Tm2]  "Tm2"
  [polyvals] -> Selector1/1
  Constant/1 -> Selector1/2
  Selector1/1 -> [Tm1]  "Tm1"
  [x] -> Product/1
  [Tm1] -> Product/2
  Product/1 -> Gain/1
  Gain/1 -> Add/1
  [Tm2] -> Add/2
  Add/1 -> polyval/1  "if.polyval"

== system simQuadrotor/Controller/Disturbance Estimator/getDisturbance/Chebyshev Basis Functions/Chebyshev Polynomail Value Calculation/If Action Subsystem1 ==
  x : Inport
  N : Inport  Port=2
  Action Port : ActionPort  PropagateVarSize=During execution  ActionType=else
  Bias1 : Bias  Bias=-1
  Data Type Conversion : DataTypeConversion
  Math Function : Math  Operator=pow  OutputSignalType=real  SaturateOnIntegerOverflow=on
  polval : Outport
  wires:
  x/1 -> Math Function/1
  N/1 -> Bias1/1  "else.N"
  Math Function/1 -> polval/1  "else.polyval"
  Data Type Conversion/1 -> Math Function/2
  Bias1/1 -> Data Type Conversion/1

== system simQuadrotor/Controller/Disturbance Estimator/getDisturbance/getDhat/getW1/Projection ==
  theta : Inport
  y : Inport  Port=2
  Thetamax : Inport  Port=3
  epsilontheta : Inport  Port=4
  Bias : Bias  Bias=1
  Bias1 : Bias  Bias=1
  Divide : Product  Inputs=*/
  Divide1 : Product  Inputs=*/
  Dot Product : DotProduct  InputSameDT=on  OutDataTypeStr=Inherit: Inherit via internal rule
  Gain : Gain  Gain=2
  Math Function : Math  Operator=square  SaturateOnIntegerOverflow=on
  Math Function1 : Math  Operator=square  SaturateOnIntegerOverflow=on
  Normalize Vector1 : vrlib/Utilities/Normalize Vector  maxzero=0
  Product{,1..3,6..7} (6 alike) : Product  RndMeth=Zero
  Product4 : Product  Multiplication=Matrix(*)  RndMeth=Zero
  Product5 : Product  Multiplication=Matrix(*)  RndMeth=Zero
  Reshape : Reshape  OutputDimensionality=Row vector (2-D)
  Reshape1 : Reshape  OutputDimensionality=Row vector (2-D)
  Sum4 : Sum  Inputs=|+-
  Sum5 : Sum  Inputs=|+-
  Switch : Switch  Criteria=u2 > Threshold
  Switch1 : Switch  Criteria=u2 > Threshold
  Proj : Outport
  wires:
  [f] -> Switch/2
  y/1 -> [y]
  Switch/1 -> Proj/1
  Product5/1 -> Switch1/2
  [y] -> Product5/2
  Sum4/1 -> Divide/1
  Math Function/1 -> Sum4/2, Product2/1
  Product4/1 -> Product3/2
  [theta] -> Reshape1/1, Product4/2
  [df] -> Reshape/1
  Reshape/1 -> Product5/1
  Reshape1/1 -> Product4/1
  theta/1 -> [theta]
  [y] -> Switch/3
  Switch1/1 -> Switch/1
  [y] -> Sum5/1
  Product/1 -> Product1/1
  [y] -> Switch1/3
  Product1/1 -> Sum5/2
  Sum5/1 -> Switch1/1
  [f] -> Product1/2
  [df] -> Normalize Vector1/1
  Normalize Vector1/1 -> Dot Product/1, Product/1
  [y] -> Dot Product/2
  Dot Product/1 -> Product/2
  Thetamax/1 -> [Thetamax]
  [Thetamax] -> Math Function/1
  epsilontheta/1 -> [epsilontheta]
  [epsilontheta] -> Product2/2
  Product2/1 -> Divide/2
  Divide/1 -> [f]
  Product3/1 -> Sum4/1
  Bias/1 -> Product3/1
  [epsilontheta] -> Bias/1
  [epsilontheta] -> Bias1/1, Product6/1
  Bias1/1 -> Gain/1
  Gain/1 -> Divide1/1
  [Thetamax] -> Math Function1/1
  Math Function1/1 -> Product6/2
  Product6/1 -> Divide1/2
  Product7/1 -> [df]
  [theta] -> Product7/1
  Divide1/1 -> Product7/2

== system simQuadrotor/Controller/Disturbance Estimator/getDisturbance/getDhat/getW2/Projection ==
  theta : Inport
  y : Inport  Port=2
  Thetamax : Inport  Port=3
  epsilontheta : Inport  Port=4
  Bias : Bias  Bias=1
  Bias1 : Bias  Bias=1
  Divide : Product  Inputs=*/
  Divide1 : Product  Inputs=*/
  Dot Product : DotProduct  InputSameDT=on  OutDataTypeStr=Inherit: Inherit via internal rule
  Gain : Gain  Gain=2
  Math Function : Math  Operator=square  SaturateOnIntegerOverflow=on
  Math Function1 : Math  Operator=square  SaturateOnIntegerOverflow=on
  Normalize Vector1 : vrlib/Utilities/Normalize Vector  maxzero=0
  Product{,1..3,6..7} (6 alike) : Product  RndMeth=Zero
  Product4 : Product  Multiplication=Matrix(*)  RndMeth=Zero
  Product5 : Product  Multiplication=Matrix(*)  RndMeth=Zero
  Reshape : Reshape  OutputDimensionality=Row vector (2-D)
  Reshape1 : Reshape  OutputDimensionality=Row vector (2-D)
  Sum4 : Sum  Inputs=|+-
  Sum5 : Sum  Inputs=|+-
  Switch : Switch  Criteria=u2 > Threshold
  Switch1 : Switch  Criteria=u2 > Threshold
  Proj : Outport
  wires:
  Divide1/1 -> Product7/2
  [theta] -> Product7/1
  Product7/1 -> [df]
  Product6/1 -> Divide1/2
  Math Function1/1 -> Product6/2
  [Thetamax] -> Math Function1/1
  Gain/1 -> Divide1/1
  Bias1/1 -> Gain/1
  [epsilontheta] -> Product6/1, Bias1/1
  [epsilontheta] -> Bias/1
  Bias/1 -> Product3/1
  Product3/1 -> Sum4/1
  Divide/1 -> [f]
  Product2/1 -> Divide/2
  [epsilontheta] -> Product2/2
  epsilontheta/1 -> [epsilontheta]
  [Thetamax] -> Math Function/1
  Thetamax/1 -> [Thetamax]
  Dot Product/1 -> Product/2
  [y] -> Dot Product/2
  Normalize Vector1/1 -> Product/1, Dot Product/1
  [df] -> Normalize Vector1/1
  [f] -> Product1/2
  Sum5/1 -> Switch1/1
  Product1/1 -> Sum5/2
  [y] -> Switch1/3
  Product/1 -> Product1/1
  [y] -> Sum5/1
  Switch1/1 -> Switch/1
  [y] -> Switch/3
  theta/1 -> [theta]
  Reshape1/1 -> Product4/1
  Reshape/1 -> Product5/1
  [df] -> Reshape/1
  [theta] -> Product4/2, Reshape1/1
  Product4/1 -> Product3/2
  Math Function/1 -> Product2/1, Sum4/2
  Sum4/1 -> Divide/1
  [y] -> Product5/2
  Product5/1 -> Switch1/2
  Switch/1 -> Proj/1
  y/1 -> [y]
  [f] -> Switch/2

== system simQuadrotor/Controller/Disturbance Estimator/getDisturbance/getDhat/getW3/Projection ==
  theta : Inport
  y : Inport  Port=2
  Thetamax : Inport  Port=3
  epsilontheta : Inport  Port=4
  Bias : Bias  Bias=1
  Bias1 : Bias  Bias=1
  Divide : Product  Inputs=*/
  Divide1 : Product  Inputs=*/
  Dot Product : DotProduct  InputSameDT=on  OutDataTypeStr=Inherit: Inherit via internal rule
  Gain : Gain  Gain=2
  Math Function : Math  Operator=square  SaturateOnIntegerOverflow=on
  Math Function1 : Math  Operator=square  SaturateOnIntegerOverflow=on
  Normalize Vector1 : vrlib/Utilities/Normalize Vector  maxzero=0
  Product{,1..3,6..7} (6 alike) : Product  RndMeth=Zero
  Product4 : Product  Multiplication=Matrix(*)  RndMeth=Zero
  Product5 : Product  Multiplication=Matrix(*)  RndMeth=Zero
  Reshape : Reshape  OutputDimensionality=Row vector (2-D)
  Reshape1 : Reshape  OutputDimensionality=Row vector (2-D)
  Sum4 : Sum  Inputs=|+-
  Sum5 : Sum  Inputs=|+-
  Switch : Switch  Criteria=u2 > Threshold
  Switch1 : Switch  Criteria=u2 > Threshold
  Proj : Outport
  wires:
  [f] -> Switch/2
  y/1 -> [y]
  Switch/1 -> Proj/1
  Product5/1 -> Switch1/2
  [y] -> Product5/2
  Sum4/1 -> Divide/1
  Math Function/1 -> Sum4/2, Product2/1
  Product4/1 -> Product3/2
  [theta] -> Reshape1/1, Product4/2
  [df] -> Reshape/1
  Reshape/1 -> Product5/1
  Reshape1/1 -> Product4/1
  theta/1 -> [theta]
  [y] -> Switch/3
  Switch1/1 -> Switch/1
  [y] -> Sum5/1
  Product/1 -> Product1/1
  [y] -> Switch1/3
  Product1/1 -> Sum5/2
  Sum5/1 -> Switch1/1
  [f] -> Product1/2
  [df] -> Normalize Vector1/1
  Normalize Vector1/1 -> Dot Product/1, Product/1
  [y] -> Dot Product/2
  Dot Product/1 -> Product/2
  Thetamax/1 -> [Thetamax]
  [Thetamax] -> Math Function/1
  epsilontheta/1 -> [epsilontheta]
  [epsilontheta] -> Product2/2
  Product2/1 -> Divide/2
  Divide/1 -> [f]
  Product3/1 -> Sum4/1
  Bias/1 -> Product3/1
  [epsilontheta] -> Bias/1
  [epsilontheta] -> Bias1/1, Product6/1
  Bias1/1 -> Gain/1
  Gain/1 -> Divide1/1
  [Thetamax] -> Math Function1/1
  Math Function1/1 -> Product6/2
  Product6/1 -> Divide1/2
  Product7/1 -> [df]
  [theta] -> Product7/1
  Divide1/1 -> Product7/2

== system simQuadrotor/Controller/FTC Controller/SingleProp Compensation/PD-control for Reduced Attitude-Bullo/getRedAttRelatedPars/DCM E to B ==
  phithetapsi : Inport
  Create 3x3 Matrix : aerolibutil/Create 3x3 Matrix
  Fcn11 : Fcn  Expr=u(5)*u(6)
  Fcn12 : Fcn  Expr=u(3)*u(5)
  Fcn13 : Fcn  Expr=-u(2)
  Fcn21 : Fcn  Expr=u(1)*u(2)*u(6)-u(4)*u(3)
  Fcn22 : Fcn  Expr=u(1)*u(2)*u(3)+u(4)*u(6)
  Fcn23 : Fcn  Expr=u(1)*u(5)
  Fcn31 : Fcn  Expr=u(4)*u(2)*u(6)+u(1)*u(3)
  Fcn32 : Fcn  Expr=u(4)*u(2)*u(3)-u(1)*u(6)
  Fcn33 : Fcn  Expr=u(4)*u(5)
  Mux : Mux  Inputs=2
  sincos : Trigonometry  Operator=sincos
  CB_E : Outport
  wires:
  Create 3x3 Matrix/1 -> CB_E/1  "CB_E"
  phithetapsi/1 -> sincos/1  "phithetapsi"
  Fcn33/1 -> Create 3x3 Matrix/9
  Fcn32/1 -> Create 3x3 Matrix/8
  Fcn23/1 -> Create 3x3 Matrix/6
  Fcn22/1 -> Create 3x3 Matrix/5
  Fcn31/1 -> Create 3x3 Matrix/7
  Fcn21/1 -> Create 3x3 Matrix/4
  Fcn13/1 -> Create 3x3 Matrix/3
  Fcn12/1 -> Create 3x3 Matrix/2
  Fcn11/1 -> Create 3x3 Matrix/1
  Mux/1 -> Fcn21/1, Fcn13/1, Fcn12/1, Fcn11/1, Fcn22/1, Fcn23/1, Fcn31/1, Fcn33/1, Fcn32/1
  sincos/2 -> Mux/2
  sincos/1 -> Mux/1

== system simQuadrotor/Controller/FTC Controller/SingleProp Compensation/PD-control for Reduced Attitude-Bullo/getRedAttRelatedPars/DCM E to B1 ==
  phithetapsi : Inport
  Create 3x3 Matrix : aerolibutil/Create 3x3 Matrix
  Fcn11 : Fcn  Expr=u(5)*u(6)
  Fcn12 : Fcn  Expr=u(3)*u(5)
  Fcn13 : Fcn  Expr=-u(2)
  Fcn21 : Fcn  Expr=u(1)*u(2)*u(6)-u(4)*u(3)
  Fcn22 : Fcn  Expr=u(1)*u(2)*u(3)+u(4)*u(6)
  Fcn23 : Fcn  Expr=u(1)*u(5)
  Fcn31 : Fcn  Expr=u(4)*u(2)*u(6)+u(1)*u(3)
  Fcn32 : Fcn  Expr=u(4)*u(2)*u(3)-u(1)*u(6)
  Fcn33 : Fcn  Expr=u(4)*u(5)
  Mux : Mux  Inputs=2
  sincos : Trigonometry  Operator=sincos
  CB_E : Outport
  wires:
  Create 3x3 Matrix/1 -> CB_E/1  "CB_E"
  phithetapsi/1 -> sincos/1  "phithetapsi"
  Fcn33/1 -> Create 3x3 Matrix/9
  Fcn32/1 -> Create 3x3 Matrix/8
  Fcn23/1 -> Create 3x3 Matrix/6
  Fcn22/1 -> Create 3x3 Matrix/5
  Fcn31/1 -> Create 3x3 Matrix/7
  Fcn21/1 -> Create 3x3 Matrix/4
  Fcn13/1 -> Create 3x3 Matrix/3
  Fcn12/1 -> Create 3x3 Matrix/2
  Fcn11/1 -> Create 3x3 Matrix/1
  Mux/1 -> Fcn21/1, Fcn13/1, Fcn12/1, Fcn11/1, Fcn22/1, Fcn23/1, Fcn31/1, Fcn33/1, Fcn32/1
  sincos/2 -> Mux/2
  sincos/1 -> Mux/1

== system simQuadrotor/Controller/FTC Controller/SingleProp Compensation/PD-control for Reduced Attitude-Bullo/getRedAttRelatedPars/getDistance ==
  q : Inport
  pi0 : Inport  Port=2
  3x3 Cross Product1 : aerolibutil/3x3 Cross Product
  Trigonometric Function : Trigonometry  Operator=asin
  vectorNorm : Subsystem
  dist_pi0_q : Outport
  wires:
  vectorNorm/1(vNorm) -> Trigonometric Function/1
  Trigonometric Function/1 -> [dist_pi0_q]
  q/1 -> [q]
  pi0/1 -> [pi0]
  [dist_pi0_q] -> dist_pi0_q/1
  3x3 Cross Product1/1 -> vectorNorm/1(v)
  [pi0] -> 3x3 Cross Product1/1
  [q] -> 3x3 Cross Product1/2

== system simQuadrotor/Controller/FTC Controller/SingleProp Compensation/PD-control for Reduced Attitude-Bullo/getRedAttRelatedPars/vectorNorm ==
  v : Inport
  Math Function4 : Math  Operator=transpose  SaturateOnIntegerOverflow=on
  Product8 : Product  Multiplication=Matrix(*)  RndMeth=Zero
  Sqrt1 : Sqrt  SaturateOnIntegerOverflow=on
  vNorm : Outport
  wires:
  Math Function4/1 -> Product8/1
  Product8/1 -> Sqrt1/1
  v/1 -> Math Function4/1, Product8/2
  Sqrt1/1 -> vNorm/1

== system simQuadrotor/Controller/FTC Controller/SingleProp Compensation/PD-control for Reduced Attitude-Bullo/getRedAttRelatedPars/vectorNorm1 ==
  v : Inport
  Math Function4 : Math  Operator=transpose  SaturateOnIntegerOverflow=on
  Product8 : Product  Multiplication=Matrix(*)  RndMeth=Zero
  Sqrt1 : Sqrt  SaturateOnIntegerOverflow=on
  vNorm : Outport
  wires:
  Sqrt1/1 -> vNorm/1
  v/1 -> Product8/2, Math Function4/1
  Product8/1 -> Sqrt1/1
  Math Function4/1 -> Product8/1

== system simQuadrotor/Controller/FTC Controller/SingleProp Compensation/PD-control for Reduced Attitude-Bullo/getRedAttRelatedPars/vectorNorm2 ==
  v : Inport
  Math Function4 : Math  Operator=transpose  SaturateOnIntegerOverflow=on
  Product8 : Product  Multiplication=Matrix(*)  RndMeth=Zero
  Sqrt1 : Sqrt  SaturateOnIntegerOverflow=on
  vNorm : Outport
  wires:
  Sqrt1/1 -> vNorm/1
  v/1 -> Product8/2, Math Function4/1
  Product8/1 -> Sqrt1/1
  Math Function4/1 -> Product8/1

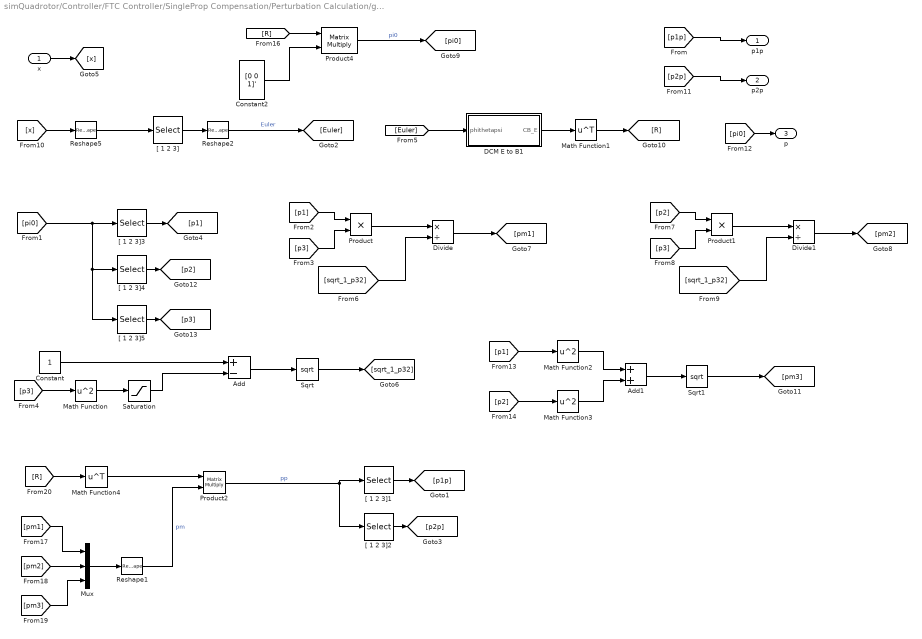
== system simQuadrotor/Controller/FTC Controller/SingleProp Compensation/Perturbation Calculation/getStates/calcParameters ==
  x : Inport
  Add : Sum  Inputs=+-
  Add1 : Sum
  Constant : Constant
  Constant2 : Constant  Value=[0 0 1]'  VectorParams1D=off
  DCM E to B1 : Subsystem
  Divide : Product  Inputs=*/
  Divide1 : Product  Inputs=*/
  Math Function : Math  Operator=square  SaturateOnIntegerOverflow=on
  Math Function1 : Math  Operator=transpose  SaturateOnIntegerOverflow=on
  Math Function2 : Math  Operator=square  SaturateOnIntegerOverflow=on
  Math Function3 : Math  Operator=square  SaturateOnIntegerOverflow=on
  Math Function4 : Math  Operator=transpose  SaturateOnIntegerOverflow=on
  Mux : Mux  Inputs=3
  Product : Product
  Product1 : Product
  Product2 : Product  Multiplication=Matrix(*)
  Product4 : Product  Multiplication=Matrix(*)  RndMeth=Zero
  Reshape1 : Reshape  OutputDimensionality=Column vector (2-D)
  Reshape2 : Reshape  OutputDimensionality=Column vector (2-D)
  Reshape5 : Reshape  OutputDimensionality=Column vector (2-D)
  Saturation : Saturate  UpperLimit=0.999999  LowerLimit=0
  Sqrt : Sqrt  SaturateOnIntegerOverflow=on
  Sqrt1 : Sqrt  SaturateOnIntegerOverflow=on
  "[ 1 2 3]" : Selector  NumberOfDimensions=2  InputPortWidth=3  IndexOptions=Index vector (dialog),Index vector (dialog)  Indices=[1 2 3],1  OutputSizes=1,1
  "[ 1 2 3]1" : Selector  InputPortWidth=3
  "[ 1 2 3]2" : Selector  InputPortWidth=3  Indices=2
  "[ 1 2 3]3" : Selector  InputPortWidth=3
  "[ 1 2 3]4" : Selector  InputPortWidth=3  Indices=2
  "[ 1 2 3]5" : Selector  InputPortWidth=3  Indices=3
  p1p : Outport
  p2p : Outport  Port=2
  p : Outport  Port=3
  wires:
  [pi0] -> p/1
  Saturation/1 -> Add/2
  [p2p] -> p2p/1
  x/1 -> [x]
  DCM E to B1/1(CB_E) -> Math Function1/1
  [Euler] -> DCM E to B1/1(phithetapsi)
  Reshape2/1 -> [Euler]  "Euler"
  Reshape5/1 -> "[ 1 2 3]"/1
  "[ 1 2 3]"/1 -> Reshape2/1
  [x] -> Reshape5/1
  Math Function1/1 -> [R]
  Product4/1 -> [pi0]  "pi0"
  Constant2/1 -> Product4/2
  [R] -> Product4/1
  [p1p] -> p1p/1
  Product2/1 -> "[ 1 2 3]1"/1, "[ 1 2 3]2"/1  "pp"
  "[ 1 2 3]1"/1 -> [p1p]
  "[ 1 2 3]2"/1 -> [p2p]
  [p1] -> Product/1
  [p3] -> Product/2
  Add/1 -> Sqrt/1
  Math Function/1 -> Saturation/1
  Constant/1 -> Add/1
  [p3] -> Math Function/1
  Sqrt/1 -> [sqrt_1_p32]
  Divide/1 -> [pm1]
  Product/1 -> Divide/1
  [sqrt_1_p32] -> Divide/2
  [p2] -> Product1/1
  [p3] -> Product1/2
  Divide1/1 -> [pm2]
  Product1/1 -> Divide1/1
  [sqrt_1_p32] -> Divide1/2
  Add1/1 -> Sqrt1/1
  [p1] -> Math Function2/1
  [p2] -> Math Function3/1
  Math Function2/1 -> Add1/1
  Math Function3/1 -> Add1/2
  Sqrt1/1 -> [pm3]
  [pm2] -> Mux/2
  [pm3] -> Mux/3
  [pm1] -> Mux/1
  Mux/1 -> Reshape1/1
  [R] -> Math Function4/1
  Math Function4/1 -> Product2/1
  Reshape1/1 -> Product2/2  "pm"
  "[ 1 2 3]5"/1 -> [p3]
  "[ 1 2 3]4"/1 -> [p2]
  "[ 1 2 3]3"/1 -> [p1]
  [pi0] -> "[ 1 2 3]3"/1, "[ 1 2 3]4"/1, "[ 1 2 3]5"/1

== system simQuadrotor/Controller/FTC Controller/SingleProp Compensation/Perturbation Calculation/getStates/getDistance ==
  q : Inport
  p : Inport  Port=2
  3x3 Cross Product1 : aerolibutil/3x3 Cross Product
  Trigonometric Function : Trigonometry  Operator=asin
  vectorNorm : Subsystem
  dist : Outport
  wires:
  vectorNorm/1(vNorm) -> Trigonometric Function/1
  Trigonometric Function/1 -> [dist_pi0_q]
  q/1 -> [q]
  p/1 -> [pi0]
  [dist_pi0_q] -> dist/1
  3x3 Cross Product1/1 -> vectorNorm/1(v)
  [pi0] -> 3x3 Cross Product1/1
  [q] -> 3x3 Cross Product1/2

== system simQuadrotor/Controller/Nominal Controller/PD-Attitude Control with wB_IB/get eR/get Omega(R) RBAC/get a ==
  C : Inport
  11 : Selector  NumberOfDimensions=2  InputPortWidth=3  IndexOptions=Index vector (dialog),Index vector (dialog)  Indices=1,1  OutputSizes=1,1
  12 : Selector  NumberOfDimensions=2  InputPortWidth=3  IndexOptions=Index vector (dialog),Index vector (dialog)  Indices=1,2  OutputSizes=1,1
  13 : Selector  NumberOfDimensions=2  InputPortWidth=3  IndexOptions=Index vector (dialog),Index vector (dialog)  Indices=1,3  OutputSizes=1,1
  21 : Selector  NumberOfDimensions=2  InputPortWidth=3  IndexOptions=Index vector (dialog),Index vector (dialog)  Indices=2,1  OutputSizes=1,1
  22 : Selector  NumberOfDimensions=2  InputPortWidth=3  IndexOptions=Index vector (dialog),Index vector (dialog)  Indices=2,2  OutputSizes=1,1
  23 : Selector  NumberOfDimensions=2  InputPortWidth=3  IndexOptions=Index vector (dialog),Index vector (dialog)  Indices=2,3  OutputSizes=1,1
  31 : Selector  NumberOfDimensions=2  InputPortWidth=3  IndexOptions=Index vector (dialog),Index vector (dialog)  Indices=3,1  OutputSizes=1,1
  32 : Selector  NumberOfDimensions=2  InputPortWidth=3  IndexOptions=Index vector (dialog),Index vector (dialog)  Indices=3,2  OutputSizes=1,1
  33 : Selector  NumberOfDimensions=2  InputPortWidth=3  IndexOptions=Index vector (dialog),Index vector (dialog)  Indices=3,3  OutputSizes=1,1
  Add : Sum  Inputs=+++-
  Add1 : Sum  Inputs=+-
  Add2 : Sum  Inputs=+-
  Add3 : Sum  Inputs=+-
  Constant5 : Constant
  Divide : Product  Inputs=*/
  Gain1 : Gain  Gain=0.5
  Gain2 : Gain  Gain=2
  Gain3 : Gain
  Mux : Mux  Inputs=3
  Product : Product  RndMeth=Zero
  Trigonometric Function : Trigonometry  Operator=acos
  Trigonometric Function1 : Trigonometry
  a : Outport
  wires:
  [alpha] -> Product/2
  Product/1 -> Gain3/1
  Divide/1 -> Product/1
  Gain3/1 -> [a]  "a"
  [a] -> a/1
  Gain2/1 -> Divide/2
  Mux/1 -> Divide/1
  [sinAlpha] -> Gain2/1
  Add3/1 -> Mux/3
  Add2/1 -> Mux/2
  Add1/1 -> Mux/1
  [C21] -> Add3/2
  [C12] -> Add3/1
  [C13] -> Add2/2
  [C31] -> Add2/1
  [C32] -> Add1/2
  [C23] -> Add1/1
  Trigonometric Function1/1 -> [sinAlpha]
  [alpha] -> Trigonometric Function1/1
  Trigonometric Function/1 -> [alpha]  "alpha"
  Gain1/1 -> Trigonometric Function/1
  Add/1 -> Gain1/1
  Constant5/1 -> Add/4
  [C33] -> Add/3
  [C22] -> Add/2
  [C11] -> Add/1
  33/1 -> [C33]
  32/1 -> [C32]
  31/1 -> [C31]
  23/1 -> [C23]
  22/1 -> [C22]
  21/1 -> [C21]
  13/1 -> [C13]
  12/1 -> [C12]
  11/1 -> [C11]
  C/1 -> 11/1, 12/1, 13/1, 21/1, 22/1, 23/1, 31/1, 32/1, 33/1

== system simQuadrotor/Controller/Nominal Controller/PD-Attitude Control with wB_IB/get eR/get eR/get alpha ==
  C : Inport
  11 : Selector  NumberOfDimensions=2  InputPortWidth=3  IndexOptions=Index vector (dialog),Index vector (dialog)  Indices=1,1  OutputSizes=1,1
  22 : Selector  NumberOfDimensions=2  InputPortWidth=3  IndexOptions=Index vector (dialog),Index vector (dialog)  Indices=2,2  OutputSizes=1,1
  33 : Selector  NumberOfDimensions=2  InputPortWidth=3  IndexOptions=Index vector (dialog),Index vector (dialog)  Indices=3,3  OutputSizes=1,1
  Add : Sum  Inputs=+++-
  Constant5 : Constant
  Gain1 : Gain  Gain=0.5
  Trigonometric Function : Trigonometry  Operator=acos
  alpha : Outport
  wires:
  C/1 -> 33/1, 11/1, 22/1
  11/1 -> [C11]
  22/1 -> [C22]
  33/1 -> [C33]
  [C11] -> Add/1
  [C22] -> Add/2
  [C33] -> Add/3
  Constant5/1 -> Add/4
  Add/1 -> Gain1/1
  Gain1/1 -> Trigonometric Function/1
  Trigonometric Function/1 -> [alpha]  "alpha"
  [alpha] -> alpha/1

== system simQuadrotor/Controller/Nominal Controller/PD-control for Reduced Attitude-Bullo/getRedAttRelatedPars/getDistance/vectorNorm ==
  v : Inport
  Math Function4 : Math  Operator=transpose  SaturateOnIntegerOverflow=on
  Product8 : Product  Multiplication=Matrix(*)  RndMeth=Zero
  Sqrt1 : Sqrt  SaturateOnIntegerOverflow=on
  vNorm : Outport
  wires:
  Sqrt1/1 -> vNorm/1
  v/1 -> Product8/2, Math Function4/1
  Product8/1 -> Sqrt1/1
  Math Function4/1 -> Product8/1

== system simQuadrotor/Controller/FTC Controller/SingleProp Compensation/PD-control for Reduced Attitude-Bullo/getRedAttRelatedPars/getDistance/vectorNorm ==
  v : Inport
  Math Function4 : Math  Operator=transpose  SaturateOnIntegerOverflow=on
  Product8 : Product  Multiplication=Matrix(*)  RndMeth=Zero
  Sqrt1 : Sqrt  SaturateOnIntegerOverflow=on
  vNorm : Outport
  wires:
  Math Function4/1 -> Product8/1
  Product8/1 -> Sqrt1/1
  v/1 -> Math Function4/1, Product8/2
  Sqrt1/1 -> vNorm/1

== system simQuadrotor/Controller/FTC Controller/SingleProp Compensation/Perturbation Calculation/getStates/calcParameters/DCM E to B1 ==
  phithetapsi : Inport
  Create 3x3 Matrix : aerolibutil/Create 3x3 Matrix
  Fcn11 : Fcn  Expr=u(5)*u(6)
  Fcn12 : Fcn  Expr=u(3)*u(5)
  Fcn13 : Fcn  Expr=-u(2)
  Fcn21 : Fcn  Expr=u(1)*u(2)*u(6)-u(4)*u(3)
  Fcn22 : Fcn  Expr=u(1)*u(2)*u(3)+u(4)*u(6)
  Fcn23 : Fcn  Expr=u(1)*u(5)
  Fcn31 : Fcn  Expr=u(4)*u(2)*u(6)+u(1)*u(3)
  Fcn32 : Fcn  Expr=u(4)*u(2)*u(3)-u(1)*u(6)
  Fcn33 : Fcn  Expr=u(4)*u(5)
  Mux : Mux  Inputs=2
  sincos : Trigonometry  Operator=sincos
  CB_E : Outport
  wires:
  sincos/1 -> Mux/1
  sincos/2 -> Mux/2
  Mux/1 -> Fcn32/1, Fcn33/1, Fcn31/1, Fcn23/1, Fcn22/1, Fcn11/1, Fcn12/1, Fcn13/1, Fcn21/1
  Fcn11/1 -> Create 3x3 Matrix/1
  Fcn12/1 -> Create 3x3 Matrix/2
  Fcn13/1 -> Create 3x3 Matrix/3
  Fcn21/1 -> Create 3x3 Matrix/4
  Fcn31/1 -> Create 3x3 Matrix/7
  Fcn22/1 -> Create 3x3 Matrix/5
  Fcn23/1 -> Create 3x3 Matrix/6
  Fcn32/1 -> Create 3x3 Matrix/8
  Fcn33/1 -> Create 3x3 Matrix/9
  phithetapsi/1 -> sincos/1  "phithetapsi"
  Create 3x3 Matrix/1 -> CB_E/1  "CB_E"

== system simQuadrotor/Controller/FTC Controller/SingleProp Compensation/Perturbation Calculation/getStates/getDistance/vectorNorm ==
  v : Inport
  Math Function4 : Math  Operator=transpose  SaturateOnIntegerOverflow=on
  Product8 : Product  Multiplication=Matrix(*)  RndMeth=Zero
  Sqrt1 : Sqrt  SaturateOnIntegerOverflow=on
  vNorm : Outport
  wires:
  Math Function4/1 -> Product8/1
  Product8/1 -> Sqrt1/1
  v/1 -> Math Function4/1, Product8/2
  Sqrt1/1 -> vNorm/1
